simulink model "CryoDetMultiChan_CMB"  (R2016b)
settings: Solver=ode45  StartTime=0.0  StopTime=1000e-6  MaxStep=Tclk/4  RelTol=1e-3
values from neighbouring files (symbols this model uses):
  ds_axi = 16    [setupCryoFPGA_CMB.m]
  Fclk = Fadc    (= 307200000)    [setupCryoFPGA.m]    (also in setupCryoFPGA_CMB.m; setupCryoFPGAorig.m = 312500000)
  notch = tf( [1 a*wNotch/Q wNotch^2], [1 wNotch/Q wNotch^2])    [setupCryoFPGA.m]    (also in setupCryoFPGA_CMB.m; setupCryoFPGAorig.m)
  notch2 = tf( [1 a*wNotch/Q wNotch^2], [1 wNotch/Q wNotch^2])    [setupCryoFPGA.m]    (also in setupCryoFPGA_CMB.m; setupCryoFPGAorig.m)
  notch3 = tf( [1 a*wNotch/Q wNotch^2], [1 wNotch/Q wNotch^2])    [setupCryoFPGA.m]    (also in setupCryoFPGA_CMB.m; setupCryoFPGAorig.m)
  notch4 = tf( [1 a*wNotch/Q wNotch^2], [1 wNotch/Q wNotch^2])    [setupCryoFPGA.m]    (also in setupCryoFPGA_CMB.m; setupCryoFPGAorig.m)
  Tclk = 1/Fclk    (= 3.25520833333e-09)    [setupCryoFPGA.m]    (also in setupCryoFPGA_CMB.m; setupCryoFPGAorig.m = 3.2e-09)
  Ts = 1/Fadc    (= 3.25520833333e-09)    [setupCryoFPGA.m]    (also in setupCryoFPGA_CMB.m; setupCryoFPGAorig.m = 3.2e-09)
undefined symbols (not defined in the file or in its folder): AXI4, i, Lite, xlipgetpartsetting
libraries: xbsIndex_r4 x2077, CryoDetLib x32, hdlsllib x6, simulink x3
(part 1 of 15)
settings Model: Creator=ssmith  LastModifiedBy=jedu
settings DataIOCC: LimitDataPoints=on  SaveFormat=Array
settings OptimizationCC: BlockReduction=off  BooleanDataType=off  LifeSpan=inf
settings DebuggingCC: SaveWithParameterizedLinksMsg=none  UnderspecifiedInitializationDetection=Classic  MergeDetectMultiDrivingBlocksExec=none  SignalResolutionControl=TryResolveAllWithWarning  AllowSymbolicDim=off  SFUnexpectedBacktrackingDiag=warning  SFNoUnconditionalDefaultTransitionDiag=warning  SFExecutionAtInitializationDiag=none
settings HardwareCC: ProdBitPerPointer=32  ProdBitPerSizeT=32  ProdBitPerPtrDiffT=32  ProdLargestAtomicFloat=None  ProdIntDivRoundTo=Undefined  ProdEndianess=Unspecified  ProdWordSize=32  ProdHWDeviceType=32-bit Generic  TargetUnknown=on
settings ModelReferenceCC: PropagateSignalLabelsOutOfModel=off
settings GRTTargetCC: TargetLangStandard=C89/C90 (ANSI)  GeneratePreprocessorConditionals=Disable all
settings ConfigComp: CovMetricSettings=dw  CovHtmlReporting=on  CovSaveCumulativeToWorkspaceVar=on  CovSaveSingleToWorkspaceVar=on  CovExternalEMLEnable=off  CovSFcnEnable=off

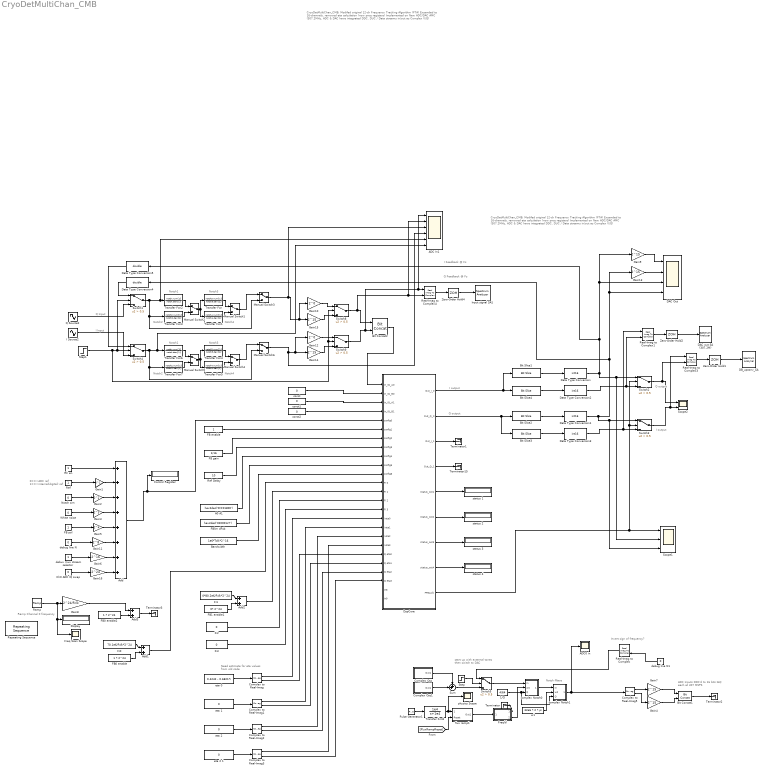
== system CryoDetMultiChan_CMB ==
  note: Notch1
  note: 0==>ADC ref
      | 1==>internal(digital) ref
  note: Q output
  note: I output
  note: Q output
  note: I output
  note: Q Feedback @ Fs
  note: I Feedback @ Fs
  note: Need estimate for eta values
      | from old code
  note: Invert sign of frequency?
  note: Notch filters
  note: start up with external tones
      | then switch to DAC
  note: CryoDetMultiChan_CMB:
      |
      | Modifed original 12-ch Frequency Tracking Algorithm (FTA)
      | Expanded to 16-channels, removed eta calculation (now prog registers)
      | Implemented on New ADC/DAC AMC (307.2MHz, ADC & DAC have integrated DDC, DUC / Data streams in/out as Complex (I/Q)
  note: ADC Inputs DDC'd to
      | 16 bits I&Q each at 307 MSPS
  note: Q Input
  note: I Input
  note: Notch2
  note: Notch3
  note: Notch4
  note: Notch1
  note: Notch2
  note: Notch3
  note: Notch4
  note: Ramp Channel 0 frequency
  note: CryoDetMultiChan_CMB:
      |
      | Modifed original 12-ch Frequency Tracking Algorithm (FTA)
      | Expanded to 16-channels, removed eta calculation (now prog registers)
      | Implemented on New ADC/DAC AMC (307.2MHz, ADC & DAC have integrated DDC, DUC / Data streams in/out as Complex (I/Q)
  1/Q : Constant  Value=4/64  SampleTime=Tclk
  A0 A1 : Constant  Value=hex2dec('FFF01800')  SampleTime=Tclk
  ADC In1 : Scope  NumInputPorts=6
  ADC0 in : Scope
  Add : Sum  Inputs=++++++++
  Add1 : Sum
  Add2 : Sum
  Add3 : Sum
  Bandwidth : Constant  Value=1e6*Tclk*2^16  SampleTime=Tclk
  Bit Concat1 : hdlsllib/HDL Operations/Bit Concat  numInputs=2
  Bit Concat2 : hdlsllib/HDL Operations/Bit Concat  numInputs=2
  Bit Slice1 : hdlsllib/HDL Operations/Bit Slice  lidx=31  ridx=16
  Bit Slice2 : hdlsllib/HDL Operations/Bit Slice  lidx=31  ridx=16
  Bit Slice3 : hdlsllib/HDL Operations/Bit Slice  lidx=15  ridx=0
  Bit Slice4 : hdlsllib/HDL Operations/Bit Slice  lidx=15  ridx=0
  Ch0 ADC IQ swap : Constant  Value=0  SampleTime=Tclk
  Complex Osc : Subsystem  mask{Freq=40e6, Ampl=0.2}
  Complex Osc1 : Subsystem  mask{Freq=50e6, Ampl=0.2}
  Complex to Real-Imag{,1..3,5} (5 alike) : ComplexToRealImag
  Control Register : Display
      settings: Format=decimal (Stored Integer)  Decimation=1000
  DAC Out : Scope  NumInputPorts=4
  DAC out SA (307.2M) : SpectrumAnalyzer
  DB_upconv_SA : SpectrumAnalyzer
  Data Type Conversion{,1..3} (4 alike) : DataTypeConversion  OutDataTypeStr=int16
  Data Type Conversion4 : DataTypeConversion  OutMin=[-0.999]  OutMax=[0.999]  OutDataTypeStr=double  RndMeth=Nearest
  Data Type Conversion5 : DataTypeConversion  OutMin=[-0.999]  OutMax=[0.999]  OutDataTypeStr=double  RndMeth=Nearest
  Display : Display
      settings: Decimation=64
  DspCore : Subsystem
  FB enable : Constant  SampleTime=Tclk
  FB gain : Constant  Value=1/16  SampleTime=Tclk
  FB pol : Constant  SampleTime=Tclk
  FB0 enable : Constant  Value=1 * 2^24  SampleTime=Tclk
  FB0 enable2 : Constant  Value=1 * 2^24  SampleTime=Tclk
  FB1 enable1 : Constant  Value=0* 2^24  SampleTime=Tclk
  FBlim dFsb : Constant  Value=hex2dec('020001c7')  SampleTime=Tclk
  Fi0 : Constant  Value=70.1e6/Fclk*2^24  SampleTime=Tclk
  Fi1 : Constant  Value=0*80.2e6/Fclk*2^24  SampleTime=Tclk
  Fi2 : Constant  Value=0  SampleTime=Tclk
  Fi3 : Constant  Value=0  SampleTime=Tclk
  Freq Scan Scope : Scope
  "Freq(t) " : Subsystem
  Gain1 : Gain  Gain=2^1
  Gain10 : Gain  Gain=2^0  OutDataTypeStr=int16  RndMeth=Nearest  SaturateOnIntegerOverflow=on
  Gain11 : Gain  Gain=2^8
  Gain12 : Gain  Gain=2^0  OutDataTypeStr=int16  RndMeth=Nearest  SaturateOnIntegerOverflow=on
  Gain{4,7,9,13..15} (6 alike) : Gain  Gain=2^15  OutDataTypeStr=int16  RndMeth=Nearest  SaturateOnIntegerOverflow=on
  Gain16 : Gain  Gain=2^24
  Gain2 : Gain  Gain=2^2
  Gain3 : Gain  Gain=2^3
  Gain5 : Gain  Gain=2^4
  Gain6 : Gain  Gain=2^16
  Gain8 : Gain  Gain=2^24/Fclk
  I Source2 : Sin  Amplitude=.999  Frequency=2*pi*70.1e6  Phase=pi/2  SampleTime=0
  Input signal SA1 : SpectrumAnalyzer
  Manual Switch{1..6} (6 alike) : ManualSwitch
  Notch sim : Constant  Value=0  SampleTime=Tclk
  Pulse Generator1 : DiscretePulseGenerator  PulseType=Time based  Amplitude=10  Period=1e-3  PhaseDelay=12e-6
  Q Source2 : Sin  Amplitude=-0.999  Frequency=2*pi*70.1e6  SampleTime=0
  RF en : Constant  SampleTime=Tclk
  Ramp : simulink/Sources/Ramp  slope=1e6/4e-6  start=0  X0=65.1e6
  Real-Imag to Complex{,1,3..4} (4 alike) : RealImagToComplex
  Ref : Constant  SampleTime=Tclk
  Ref Delay : Constant  Value=10  SampleTime=Tclk
  Repeating Sequence : simulink/Sources/Repeating Sequence  rep_seq_t="[0   5e-6  5.1e-6  8e-6 8.1e-6   11e-6 11.1e-6   14e-6 14.1e-6   17e-6 17.1e-6 20e-6 20.1e-6 23e-6 ]"  rep_seq_y="[39.24 39.24 39.49  39.49 39.64 39.64 39.74 39.74 39.84 39.84 39.99 39.99 40.24 40.24]*1e6"
  Scope1 : Scope  NumInputPorts=3
  Scope2 : Scope  NumInputPorts=2
  Step : Step  Time=2e-7  SampleTime=0
  Step1 : Step  Time=200e-9  SampleTime=0
  Sum : Sum  Inputs=++|
  Switch{1..5,8..9} (7 alike) : Switch  Criteria=u2 > Threshold  Threshold=0.5
  Terminator{,1..3,15} (5 alike) : Terminator
  Transfer Fcn : TransferFcn  Numerator=notch3.num{1}  Denominator=notch3.den{1}
  Transfer Fcn1 : TransferFcn  Numerator=notch4.num{1}  Denominator=notch4.den{1}
  Transfer Fcn2 : TransferFcn  Numerator=notch.num{1}  Denominator=notch.den{1}
  Transfer Fcn3 : TransferFcn  Numerator=notch2.num{1}  Denominator=notch2.den{1}
  Transfer Fcn4 : TransferFcn  Numerator=notch3.num{1}  Denominator=notch3.den{1}
  Transfer Fcn5 : TransferFcn  Numerator=notch4.num{1}  Denominator=notch4.den{1}
  Transfer Fcn6 : TransferFcn  Numerator=notch.num{1}  Denominator=notch.den{1}
  Transfer Fcn7 : TransferFcn  Numerator=notch2.num{1}  Denominator=notch2.den{1}
  Transfer Fcn8 : TransferFcn  Numerator=[1e4]  Denominator=[1 1e4]
  White noise : Constant  Value=0  SampleTime=Tclk
  Zero-Order Hold1 : ZeroOrderHold  SampleTime=Ts/2
  Zero-Order Hold2 : ZeroOrderHold  SampleTime=-1
  Zero-Order Hold4 : ZeroOrderHold  SampleTime=Ts
  complex Notch0 : Subsystem
  complex Notch1 : Subsystem
  const : Constant  Value=0  SampleTime=Tclk
  const1 : Constant  Value=0  SampleTime=Tclk
  const2 : Constant  Value=0  SampleTime=Tclk
  debug line N : Constant  Value=0  SampleTime=Tclk
  debug line N1 : Constant  Value=0  SampleTime=Tclk
  debux mux stream selector : Constant  SampleTime=Tclk
  eta 0 : Constant  Value=0.4242 - 0.6821*i
  eta 1 : Constant  Value=0
  "eta 2 " : Constant  Value=0
  eta 2 1 : Constant  Value=0
  flux ramp1 : Subsystem
  physics Scope : Scope
  status {1..4} (4 alike) : Display
  w1 : Constant  Value=32e6 * 2 * pi  SampleTime=Tclk
  wires:
  Add/1 -> DspCore/5(config0), Control Register/1
  FB enable/1 -> DspCore/6(config1)
  RF en/1 -> Add/1
  Ref/1 -> Gain1/1
  Notch sim/1 -> Gain2/1
  White noise/1 -> Gain3/1
  FB pol/1 -> Gain5/1
  Gain1/1 -> Add/2
  Gain2/1 -> Add/3
  Gain3/1 -> Add/4
  Gain5/1 -> Add/5
  FB gain/1 -> DspCore/7(config2)
  Ref Delay/1 -> DspCore/8(config3)
  A0 A1/1 -> DspCore/9(config4)
  FBlim dFsb/1 -> DspCore/10(config5)
  Bandwidth/1 -> DspCore/11(config6)
  Add2/1 -> DspCore/13(Fi 1)
  FB1 enable1/1 -> Add2/2
  Fi1/1 -> Add2/1
  DspCore/9(FPGAclk) -> Switch3/2, Switch2/2, Scope1/1
  DspCore/1(Out_I_0) -> Bit Slice1/1, Bit Slice4/1
  Data Type Conversion1/1 -> Data Type Conversion4/1, DAC Out/4, Gain13/1, Scope1/3, Switch3/1
  Data Type Conversion/1 -> Data Type Conversion5/1, DAC Out/3, Gain9/1, Scope1/2, Switch2/1
  DspCore/2(Out_Q_0) -> Bit Slice3/1, Bit Slice2/1
  Switch2/1 -> Real-Imag to Complex3/2, Scope2/1
  Zero-Order Hold1/1 -> DB_upconv_SA/1
  Real-Imag to Complex3/1 -> Zero-Order Hold1/1
  Bit Slice4/1 -> Data Type Conversion2/1
  Bit Slice3/1 -> Data Type Conversion3/1
  Data Type Conversion2/1 -> Real-Imag to Complex1/2, Switch2/3
  Data Type Conversion3/1 -> Real-Imag to Complex1/1, Switch3/3
  Zero-Order Hold2/1 -> DAC out SA (307.2M)/1
  Real-Imag to Complex1/1 -> Zero-Order Hold2/1
  Switch3/1 -> Real-Imag to Complex3/1, Scope2/2
  DspCore/5(status_out1) -> status 1/1
  DspCore/6(status_out2) -> status 2/1
  DspCore/7(status_out3) -> status 3/1
  DspCore/8(status_out4) -> status 4/1
  eta 1/1 -> Complex to Real-Imag1/1
  "eta 2 "/1 -> Complex to Real-Imag2/1
  Fi2/1 -> DspCore/14(Fi 2)
  Fi3/1 -> DspCore/15(Fi 3)
  Complex to Real-Imag/1 -> DspCore/16(I eta0)
  Complex to Real-Imag/2 -> DspCore/20(Q eta0)
  Complex to Real-Imag1/1 -> DspCore/17(I eta1)
  Complex to Real-Imag1/2 -> DspCore/21(Q eta1)
  eta 2 1/1 -> Complex to Real-Imag3/1
  DspCore/3(Out_I_1) -> Terminator1/1
  DspCore/4(Out_Q_1) -> Terminator15/1
  Complex to Real-Imag2/1 -> DspCore/18(I eta2)
  Complex to Real-Imag2/2 -> DspCore/22(Q eta2)
  Complex to Real-Imag3/1 -> DspCore/19(I eta3)
  Complex to Real-Imag3/2 -> DspCore/23(Q eta3)
  const/1 -> DspCore/2(In_IQ_B0)
  const1/1 -> DspCore/3(In_IQ_A1)
  const2/1 -> DspCore/4(In_IQ_B1)
  Sum/1 -> Switch5/3
  Step/1 -> Switch5/2
  complex Notch1/1(Out) -> Complex to Real-Imag5/1, ADC0 in/1
  Switch5/1 -> complex Notch0/1(In)
  Complex Osc1/1(Out1) -> Sum/2
  Complex Osc/1(Out1) -> Sum/1
  complex Notch0/1(Out) -> complex Notch1/1(In)
  "Freq(t) "/2(omega Out) -> complex Notch0/2(w0)
  w1/1 -> complex Notch1/2(w0)
  1/Q/1 -> complex Notch1/3(Q), complex Notch0/3(Q)
  flux ramp1/1(Out1) -> "Freq(t) "/1(freq in)
  "Freq(t) "/1(Freq Out) -> Terminator/1
  [FluxRampReset] -> flux ramp1/2(Reset)
  Pulse Generator1/1 -> Transfer Fcn8/1
  Transfer Fcn8/1 -> physics Scope/1, flux ramp1/1(physics)
  Real-Imag to Complex/1 -> Switch5/1
  Gain7/1 -> Bit Concat1/1
  Gain4/1 -> Bit Concat1/2
  Complex to Real-Imag5/1 -> Gain7/1
  Complex to Real-Imag5/2 -> Gain4/1
  Manual Switch1/1 -> Manual Switch3/1
  Transfer Fcn1/1 -> Manual Switch1/2
  Transfer Fcn/1 -> Manual Switch1/1
  Transfer Fcn3/1 -> Manual Switch2/2
  Transfer Fcn2/1 -> Manual Switch2/1
  Switch1/1 -> ADC In1/5, Transfer Fcn2/1, Manual Switch3/2, Transfer Fcn3/1
  Manual Switch2/1 -> Transfer Fcn/1, Transfer Fcn1/1
  Step1/1 -> Switch9/2, Switch8/2, Switch4/2, Switch1/2
  Manual Switch4/1 -> Manual Switch6/1
  Transfer Fcn5/1 -> Manual Switch4/2
  Transfer Fcn4/1 -> Manual Switch4/1
  Transfer Fcn7/1 -> Manual Switch5/2
  Transfer Fcn6/1 -> Manual Switch5/1
  Switch4/1 -> ADC In1/6, Transfer Fcn6/1, Manual Switch6/2, Transfer Fcn7/1
  Manual Switch5/1 -> Transfer Fcn4/1, Transfer Fcn5/1
  Manual Switch3/1 -> ADC In1/3, Gain10/1, Gain15/1
  Manual Switch6/1 -> ADC In1/4, Gain12/1, Gain14/1
  Q Source2/1 -> Switch1/3
  I Source2/1 -> Switch4/3
  Bit Concat1/1 -> Terminator2/1
  debug line N1/1 -> Real-Imag to Complex/2
  FB0 enable2/1 -> Add3/2
  Gain8/1 -> Add3/1
  Ramp/1 -> Freq Scan Scope/1, Display/1, Gain8/1
  FB0 enable/1 -> Add1/2
  Fi0/1 -> Add1/1
  Gain9/1 -> DAC Out/1
  Gain13/1 -> DAC Out/2
  Data Type Conversion4/1 -> Switch1/1
  Data Type Conversion5/1 -> Switch4/1
  Zero-Order Hold4/1 -> Input signal SA1/1
  Real-Imag to Complex4/1 -> Zero-Order Hold4/1
  Switch8/1 -> ADC In1/2, Real-Imag to Complex4/2, Bit Concat2/1
  Switch9/1 -> ADC In1/1, Real-Imag to Complex4/1, Bit Concat2/2
  Gain15/1 -> Switch8/3
  Gain14/1 -> Switch9/3
  Bit Concat2/1 -> DspCore/1(In_IQ_A0)
  Gain10/1 -> Switch8/1
  Gain12/1 -> Switch9/1
  Bit Slice1/1 -> Data Type Conversion/1
  Bit Slice2/1 -> Data Type Conversion1/1
  eta 0/1 -> Complex to Real-Imag/1
  Add1/1 -> DspCore/12("Fi 0 ")
  Ch0 ADC IQ swap/1 -> Gain16/1
  debux mux stream selector/1 -> Gain6/1
  debug line N/1 -> Gain11/1
  Gain11/1 -> Add/6
  Gain6/1 -> Add/7
  Gain16/1 -> Add/8
  Add3/1 -> Terminator3/1

== system CryoDetMultiChan_CMB/Complex Osc ==
  Cosine : Sin  Amplitude=Ampl  Frequency=2*pi*Freq  Phase=pi/2  SampleTime=0
  Real-Imag to Complex : RealImagToComplex
  Sine : Sin  Amplitude=Ampl  Frequency=2*pi*Freq  SampleTime=0
  Out1 : Outport
  wires:
  Real-Imag to Complex/1 -> Out1/1
  Cosine/1 -> Real-Imag to Complex/1
  Sine/1 -> Real-Imag to Complex/2

== system CryoDetMultiChan_CMB/Complex Osc1 ==
  Cosine : Sin  Amplitude=Ampl  Frequency=2*pi*Freq  Phase=pi/2  SampleTime=0
  Real-Imag to Complex : RealImagToComplex
  Sine : Sin  Amplitude=Ampl  Frequency=2*pi*Freq  SampleTime=0
  Out1 : Outport
  wires:
  Real-Imag to Complex/1 -> Out1/1
  Cosine/1 -> Real-Imag to Complex/1
  Sine/1 -> Real-Imag to Complex/2

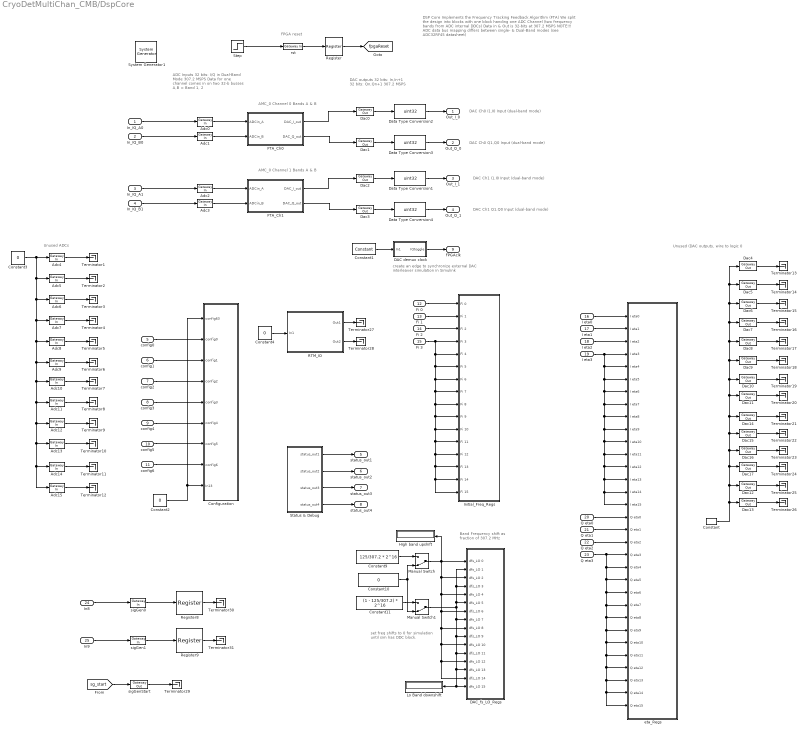
== system CryoDetMultiChan_CMB/DspCore ==
  note: AMC_0 Channel 0
      | Bands A & B
  note: Unused ADCs
  note: create an edge to synchronize external DAC interleaver simulation in Simulink
  note: DAC outputs
      | 32 bits: In,In+1
      | 32 bits: Qn,Qn+1
      | 307.2 MSPS
  note: ADC Inputs
      | 32 bits: I/Q in Dual-Band Mode
      | 307.2 MSPS
      | Data for one channel comes in on two 32-b busses A,B = Band 1, 2
  note: FPGA reset
  note: DAC Ch0 I1,I0 Input (dual-band mode)
  note: DAC Ch0 Q1,Q0 Input (dual-band mode)
  note: DSP Core
      | Implements the Frequency Tracking Feedback Algorithm (FTA)
      | We split the design into blocks with one block handing one ADC Channel
      | (two frequency bands from ADC internal DDCs)
      | Data in & Out is 32-bits at 307.2 MSPS
      |
      | NOTE!!! ADC data bus mapping differs between single- & Dual-Band modes
      | (see ADC32RF45 datasheet)
  note: DAC Ch1 I1,I0 Input (dual-band mode)
  note: DAC Ch1 Q1,Q0 Input (dual-band mode)
  note: Unused (DAC outputs, wire to logic 0
  note: set freq shifts to 0 for simulation
      | until sim has DDC block.
  note: Band Frequency shift as fraction of 307.2 MHz
  note: AMC_0 Channel 1
      | Bands A & B
  In_IQ_A0 : Inport
  In_IQ_B0 : Inport  Port=2
  In_IQ_A1 : Inport  Port=3
  In_IQ_B1 : Inport  Port=4
  config0 : Inport  Port=5
  config1 : Inport  Port=6
  config2 : Inport  Port=7
  config3 : Inport  Port=8
  config4 : Inport  Port=9
  config5 : Inport  Port=10
  config6 : Inport  Port=11
  "Fi 0 " : Inport  Port=12
  Fi 1 : Inport  Port=13
  Fi 2 : Inport  Port=14
  Fi 3 : Inport  Port=15
  I eta0 : Inport  Port=16
  I eta1 : Inport  Port=17
  I eta2 : Inport  Port=18
  I eta3 : Inport  Port=19
  Q eta0 : Inport  Port=20
  Q eta1 : Inport  Port=21
  Q eta2 : Inport  Port=22
  Q eta3 : Inport  Port=23
  In8 : Inport  Port=24
  In9 : Inport  Port=25
  " System Generator1" : xbsIndex_r4/ System Generator  Tag=genX  xilinxfamily=kintexu  part=xcku040  speed=-2-e  package=ffva1156  synthesis_tool=Vivado  clock_wrapper=Clock Enables  directory=./netlist  proj_type=Vivado  Synth_file=Vivado Synthesis Defaults  Impl_file=Vivado Implementation Defaults  testbench=off  simulink_period=Tclk  sysclk_period=Tclk*1e9  dcm_input_clock_period=10  incr_netlist=off  trim_vbits=Everywhere in SubSystem  dbl_ovrd=According to Block Masks  core_generation=According to Block Masks  run_coregen=off  deprecated_control=off  eval_field=0  block_type=sysgen
  Adc{0..15} (16 alike) : xbsIndex_r4/Gateway In  gui_display_data_type=Fixed-point  arith_type=Unsigned  n_bits=32  bin_pt=0  preci_type=Single  exp_width=8  frac_width=24  rows=1  columns=1  quantization=Truncate  overflow=Wrap  period=Ts  UseAsADC=off  ADCChannel='1'  interface=None  automatic_assignment=on  address_offset=hex2dec('00')  intf_name=''  intf_description=''  default_value=0  timing_constraint=None  locs_specified=off  LOCs={}  io_standard={}  inherit_from_input=off  hdl_port=on  dbl_ovrd=off  block_type=gatewayin
  Configuration : Subsystem
  Constant : xbsIndex_r4/Constant  const=0  gui_display_data_type=Fixed-point  arith_type=Signed (2's comp)  n_bits=32  bin_pt=0  preci_type=Single  exp_width=8  frac_width=24  explicit_period=off  period=1  equ=P=C  opselect=C  inp2=PCIN>>17  opr=+  inp1=P  carry=CIN  dbl_ovrd=off  block_type=constant
  Constant1 : xbsIndex_r4/Constant  const=0  gui_display_data_type=Boolean  arith_type=Boolean  n_bits=16  bin_pt=14  preci_type=Single  exp_width=8  frac_width=24  explicit_period=on  period=Tclk  equ=P=C  opselect=C  inp2=PCIN>>17  opr=+  inp1=P  carry=CIN  dbl_ovrd=off  block_type=constant
  Constant{2..4,10} (4 alike) : Constant  Value=0
  Constant11 : Constant  Value=(1 - 125/307.2) * 2^16
  Constant9 : Constant  Value=125/307.2 * 2^16
  DAC demux clock : Subsystem
  DAC_fs_LO_Regs : Subsystem
  Dac{0..17} (18 alike) : xbsIndex_r4/Gateway Out  inherit_from_input=on  hdl_port=on  rows=1  columns=1  UseAsDAC=off  DACChannel='1'  interface=None  automatic_assignment=on  address_offset=hex2dec('00')  intf_name=''  intf_description=''  timing_constraint=None  locs_specified=off  LOCs={}  io_standard={}  block_type=gatewayout
  Data Type Conversion{1..4} (4 alike) : DataTypeConversion  OutDataTypeStr=uint32
  FTA_Ch0 : Subsystem
  FTA_Ch1 : Subsystem
  High band upshift : Display
  Initial_Freq_Regs : Subsystem
  Lo Band downshift : Display
  Manual Switch : ManualSwitch  CurrentSetting=0
  Manual Switch1 : ManualSwitch  CurrentSetting=0
  RTM_IO : Subsystem
  Register : xbsIndex_r4/Register  init=1  rst=off  en=off  dbl_ovrd=off  block_type=register
  Register8 : xbsIndex_r4/Register  init=0  rst=off  en=off  dbl_ovrd=off  block_type=register
  Register9 : xbsIndex_r4/Register  init=0  rst=off  en=off  dbl_ovrd=off  block_type=register
  Status & Debug : Subsystem
  Step : Step  Time=300e-9  Before=1  After=0  SampleTime=0
  Terminator{1..31} (31 alike) : Terminator
  eta_Regs : Subsystem
  rst : xbsIndex_r4/Gateway In  gui_display_data_type=Boolean  arith_type=Boolean  n_bits=16  bin_pt=14  preci_type=Single  exp_width=8  frac_width=24  rows=1  columns=1  quantization="Round  (unbiased: +/- Inf)"  overflow=Saturate  period=Tclk  UseAsADC=off  ADCChannel='1'  interface=None  automatic_assignment=on  address_offset=hex2dec('00')  intf_name=''  intf_description=''  default_value=0  timing_constraint=None  locs_specified=off  LOCs={}  io_standard={}  inherit_from_input=off  hdl_port=on  dbl_ovrd=off  block_type=gatewayin
  sigGen0 : xbsIndex_r4/Gateway In  gui_display_data_type=Fixed-point  arith_type=Unsigned  n_bits=32  bin_pt=0  preci_type=Single  exp_width=8  frac_width=24  rows=1  columns=1  quantization=Truncate  overflow=Wrap  period=Ts  UseAsADC=off  ADCChannel='1'  interface=None  automatic_assignment=on  address_offset=hex2dec('00')  intf_name=''  intf_description=''  default_value=0  timing_constraint=None  locs_specified=off  LOCs={}  io_standard={}  inherit_from_input=off  hdl_port=on  dbl_ovrd=off  block_type=gatewayin
  sigGen1 : xbsIndex_r4/Gateway In  gui_display_data_type=Fixed-point  arith_type=Unsigned  n_bits=32  bin_pt=0  preci_type=Single  exp_width=8  frac_width=24  rows=1  columns=1  quantization=Truncate  overflow=Wrap  period=Ts  UseAsADC=off  ADCChannel='1'  interface=None  automatic_assignment=on  address_offset=hex2dec('00')  intf_name=''  intf_description=''  default_value=0  timing_constraint=None  locs_specified=off  LOCs={}  io_standard={}  inherit_from_input=off  hdl_port=on  dbl_ovrd=off  block_type=gatewayin
  sigGenStart : xbsIndex_r4/Gateway Out  inherit_from_input=on  hdl_port=on  rows=1  columns=1  UseAsDAC=off  DACChannel='1'  interface=None  automatic_assignment=off  address_offset=hex2dec('004')  intf_name=''  intf_description=''  timing_constraint=None  locs_specified=off  LOCs={}  io_standard={}  block_type=gatewayout
  Out_I_0 : Outport
  Out_Q_0 : Outport  Port=2
  Out_I_1 : Outport  Port=3
  Out_Q_1 : Outport  Port=4
  status_out1 : Outport  Port=5
  status_out2 : Outport  Port=6
  status_out3 : Outport  Port=7
  status_out4 : Outport  Port=8
  FPGAclk : Outport  Port=9
  tag scope: fpgaReset=global
  wires:
  In_IQ_A0/1 -> Adc0/1
  Step/1 -> rst/1
  rst/1 -> Register/1
  In_IQ_B0/1 -> Adc1/1
  Adc0/1 -> FTA_Ch0/1(ADCin_A)
  Register/1 -> [fpgaReset]
  Constant2/1 -> Configuration/1(config63), Configuration/9(In13)
  Status & Debug/1(status_out1) -> status_out1/1
  Status & Debug/2(status_out2) -> status_out2/1
  Status & Debug/3(status_out3) -> status_out3/1
  Status & Debug/4(status_out4) -> status_out4/1
  DAC demux clock/1(IQtoggle) -> FPGAclk/1
  Dac1/1 -> Data Type Conversion3/1
  FTA_Ch0/1(DAC_I_out) -> Dac0/1
  FTA_Ch0/2(DAC_Q_out) -> Dac1/1
  Data Type Conversion2/1 -> Out_I_0/1
  Dac0/1 -> Data Type Conversion2/1
  Data Type Conversion3/1 -> Out_Q_0/1
  config0/1 -> Configuration/2(config0)
  config1/1 -> Configuration/3(config1)
  config2/1 -> Configuration/4(config2)
  config4/1 -> Configuration/6(config4)
  config5/1 -> Configuration/7(config5)
  config6/1 -> Configuration/8(config6)
  In_IQ_B1/1 -> Adc3/1
  In_IQ_A1/1 -> Adc2/1
  Adc1/1 -> FTA_Ch0/2(ADCin_B)
  Adc2/1 -> FTA_Ch1/1(ADCin_A)
  Adc3/1 -> FTA_Ch1/2(ADCin_B)
  Adc4/1 -> Terminator1/1
  Adc5/1 -> Terminator2/1
  Adc6/1 -> Terminator3/1
  Adc7/1 -> Terminator4/1
  Adc8/1 -> Terminator5/1
  Adc9/1 -> Terminator6/1
  Adc10/1 -> Terminator7/1
  Adc11/1 -> Terminator8/1
  Adc12/1 -> Terminator9/1
  Adc13/1 -> Terminator10/1
  Adc14/1 -> Terminator11/1
  Adc15/1 -> Terminator12/1
  Dac3/1 -> Data Type Conversion4/1
  FTA_Ch1/1(DAC_I_out) -> Dac2/1
  FTA_Ch1/2(DAC_Q_out) -> Dac3/1
  Dac2/1 -> Data Type Conversion1/1
  Data Type Conversion1/1 -> Out_I_1/1
  Data Type Conversion4/1 -> Out_Q_1/1
  config3/1 -> Configuration/5(config3)
  Constant/1 -> Dac13/1, Dac12/1, Dac17/1, Dac16/1, Dac15/1, Dac14/1, Dac11/1, Dac10/1, Dac8/1, Dac7/1, Dac6/1, Dac5/1, Dac4/1, Dac9/1
  "Fi 0 "/1 -> Initial_Freq_Regs/1("Fi 0 ")
  Fi 1/1 -> Initial_Freq_Regs/2(Fi 1)
  Fi 2/1 -> Initial_Freq_Regs/3(Fi 2)
  Fi 3/1 -> Initial_Freq_Regs/5(Fi 4), Initial_Freq_Regs/6(Fi 5), Initial_Freq_Regs/7(Fi 6), Initial_Freq_Regs/8(Fi 7), Initial_Freq_Regs/9(Fi 8), Initial_Freq_Regs/10(Fi 9), Initial_Freq_Regs/11(Fi 10), Initial_Freq_Regs/12(Fi 11), Initial_Freq_Regs/13(Fi 12), Initial_Freq_Regs/14(Fi 13), Initial_Freq_Regs/15(Fi 14), Initial_Freq_Regs/16(Fi 15), Initial_Freq_Regs/4(Fi 3)
  I eta0/1 -> eta_Regs/1("I eta0 ")
  I eta1/1 -> eta_Regs/2(I eta1)
  I eta2/1 -> eta_Regs/3(I eta2)
  Q eta0/1 -> eta_Regs/17(Q eta0)
  Q eta1/1 -> eta_Regs/18(Q eta1)
  Q eta2/1 -> eta_Regs/19(Q eta2)
  Dac4/1 -> Terminator13/1
  Constant3/1 -> Adc5/1, Adc6/1, Adc7/1, Adc8/1, Adc9/1, Adc10/1, Adc11/1, Adc12/1, Adc13/1, Adc14/1, Adc15/1, Adc4/1
  Dac5/1 -> Terminator14/1
  Dac6/1 -> Terminator15/1
  Dac7/1 -> Terminator16/1
  Dac8/1 -> Terminator17/1
  Dac9/1 -> Terminator18/1
  Dac10/1 -> Terminator19/1
  Dac11/1 -> Terminator20/1
  Dac14/1 -> Terminator21/1
  Dac15/1 -> Terminator22/1
  Dac16/1 -> Terminator23/1
  Dac17/1 -> Terminator24/1
  Dac12/1 -> Terminator25/1
  Dac13/1 -> Terminator26/1
  Manual Switch/1 -> DAC_fs_LO_Regs/1("dfs_LO 0 "), DAC_fs_LO_Regs/3(dfs_LO 2), DAC_fs_LO_Regs/5(dfs_LO 4), DAC_fs_LO_Regs/7(dfs_LO 6), DAC_fs_LO_Regs/9(dfs_LO 8), DAC_fs_LO_Regs/11(dfs_LO 10), DAC_fs_LO_Regs/13(dfs_LO 12), DAC_fs_LO_Regs/15(dfs_LO 14), High band upshift/1
  Constant9/1 -> Manual Switch/1
  Constant10/1 -> Manual Switch/2, Manual Switch1/2
  Constant11/1 -> Manual Switch1/1
  Manual Switch1/1 -> DAC_fs_LO_Regs/8(dfs_LO 7), DAC_fs_LO_Regs/10(dfs_LO 9), DAC_fs_LO_Regs/12(dfs_LO 11), DAC_fs_LO_Regs/14(dfs_LO 13), DAC_fs_LO_Regs/16(dfs_LO 15), Lo Band downshift/1, DAC_fs_LO_Regs/6(dfs_LO 5), DAC_fs_LO_Regs/4(dfs_LO 3), DAC_fs_LO_Regs/2(dfs_LO 1)
  I eta3/1 -> eta_Regs/5(I eta4), eta_Regs/6(I eta5), eta_Regs/7(I eta6), eta_Regs/8(I eta7), eta_Regs/9(I eta8), eta_Regs/10(I eta9), eta_Regs/11(I eta10), eta_Regs/12(I eta11), eta_Regs/13(I eta12), eta_Regs/14(I eta13), eta_Regs/15(I eta14), eta_Regs/16(I eta15), eta_Regs/4(I eta3)
  Q eta3/1 -> eta_Regs/21(Q eta4), eta_Regs/22(Q eta5), eta_Regs/23(Q eta6), eta_Regs/24(Q eta7), eta_Regs/25(Q eta8), eta_Regs/26(Q eta9), eta_Regs/27(Q eta10), eta_Regs/28(Q eta11), eta_Regs/29(Q eta12), eta_Regs/30(Q eta13), eta_Regs/31(Q eta14), eta_Regs/32(Q eta15), eta_Regs/20(Q eta3)
  Constant4/1 -> RTM_IO/1(In1)
  RTM_IO/1(Out1) -> Terminator27/1
  RTM_IO/2(Out2) -> Terminator28/1
  Constant1/1 -> DAC demux clock/1(In1)
  In8/1 -> sigGen0/1
  sigGen0/1 -> Register8/1
  In9/1 -> sigGen1/1
  sigGen1/1 -> Register9/1
  sigGenStart/1 -> Terminator29/1
  [sg_start] -> sigGenStart/1
  Register8/1 -> Terminator30/1
  Register9/1 -> Terminator31/1

== system CryoDetMultiChan_CMB/Freq(t)  ==
  freq in : Inport
  Afm : Constant  Value=0.25e6
  Gain : Gain  Gain=2*pi
  Product : Product
  Ramp 0-1 : simulink/Sources/Repeating Sequence  rep_seq_t=[0 100e-6]  rep_seq_y=[0 1]
  Sine Wave Function : Sin  TimeSource=Use external signal  Frequency=2*pi  SampleTime=0
  Sum1 : Sum  Inputs=++|
  Freq Out : Outport
  omega Out : Outport  Port=2
  wires:
  Sum1/1 -> Gain/1, Freq Out/1
  Product/1 -> Sine Wave Function/1
  Ramp 0-1/1 -> Product/1
  Afm/1 -> Product/2
  Gain/1 -> omega Out/1
  Sine Wave Function/1 -> Sum1/2
  freq in/1 -> Sum1/1

== system CryoDetMultiChan_CMB/complex Notch0 ==
  In : Inport
  w0 : Inport  Port=2
  Q : Inport  Port=3
  Complex to Real-Imag : ComplexToRealImag
  Real-Imag to Complex : RealImagToComplex
  imNotch : Subsystem
  reNotch : Subsystem
  Out : Outport
  wires:
  w0/1 -> reNotch/2(w0), imNotch/2(w0)
  In/1 -> Complex to Real-Imag/1
  Q/1 -> imNotch/3(1/Q), reNotch/3(1/Q)
  Complex to Real-Imag/1 -> reNotch/1(In)
  reNotch/1(outt) -> Real-Imag to Complex/1
  imNotch/1(outt) -> Real-Imag to Complex/2
  Complex to Real-Imag/2 -> imNotch/1(In)
  Real-Imag to Complex/1 -> Out/1

== system CryoDetMultiChan_CMB/complex Notch1 ==
  In : Inport
  w0 : Inport  Port=2
  Q : Inport  Port=3
  Complex to Real-Imag : ComplexToRealImag
  Real-Imag to Complex : RealImagToComplex
  imNotch : Subsystem
  reNotch : Subsystem
  Out : Outport
  wires:
  w0/1 -> reNotch/2(w0), imNotch/2(w0)
  In/1 -> Complex to Real-Imag/1
  Q/1 -> imNotch/3(1/Q), reNotch/3(1/Q)
  Complex to Real-Imag/1 -> reNotch/1(In)
  reNotch/1(outt) -> Real-Imag to Complex/1
  imNotch/1(outt) -> Real-Imag to Complex/2
  Complex to Real-Imag/2 -> imNotch/1(In)
  Real-Imag to Complex/1 -> Out/1

== system CryoDetMultiChan_CMB/flux ramp1 ==
  note: Simulate flux-ramp modulated center frequency of notch
      | with reset from flux ramp reset
  physics : Inport
  Reset : Inport  Port=2
  Add : Sum  Inputs=++|
  Add4 : Sum
  F1 : Constant  Value=0 * 307.2e6 / 16 / 16
  F3 : Constant  Value=64e6
  Integrator : Integrator  ExternalReset=rising
  Resonator w Flux Ramp Scope : Scope
  Resonator w Flux Ramp Scope1 : Scope
  Sine Wave : Sin  TimeSource=Use external signal  Amplitude=0.1e6  Frequency=2*pi  SampleTime=0
  Out1 : Outport
  wires:
  Add4/1 -> Resonator w Flux Ramp Scope/1, Out1/1
  F3/1 -> Add4/2
  F1/1 -> Integrator/1
  Reset/1 -> Integrator/2
  Sine Wave/1 -> Add4/1
  Integrator/1 -> Add/2
  Add/1 -> Resonator w Flux Ramp Scope1/1, Sine Wave/1
  physics/1 -> Add/1

== system CryoDetMultiChan_CMB/DspCore/Configuration ==
  note: Frequencies in phase increment per clock
      | where 2^16 = 2 pi
  note: initial frequencies
  note: Configuration Registers
  note: Command Register
  note: Break out bits from Control Register (Config reg 0)
  note: Bandwidth in phase increment per clock
      | where 2^16 = 2 pi e.g 4.6875KHz/count
  config63 : Inport
  config0 : Inport  Port=2
  config1 : Inport  Port=3
  config2 : Inport  Port=4
  config3 : Inport  Port=5
  config4 : Inport  Port=6
  config5 : Inport  Port=7
  config6 : Inport  Port=8
  In13 : Inport  Port=9
  BitBasher : xbsIndex_r4/BitBasher  bitexpr=b={a[24]}  display_expr=off  sr_1=b  arith_type1=Unsigned  bin_pt1=0  sr_2=2  arith_type2=Unsigned  bin_pt2=0  sr_3=3  arith_type3=Unsigned  bin_pt3=0  sr_4=4  arith_type4=Unsigned  bin_pt4=0  dbl_ovrd=off  block_type=bitbasher
  BitBasher1 : xbsIndex_r4/BitBasher  bitexpr=b={a[25]}  display_expr=off  sr_1=b  arith_type1=Unsigned  bin_pt1=0  sr_2=2  arith_type2=Unsigned  bin_pt2=0  sr_3=3  arith_type3=Unsigned  bin_pt3=0  sr_4=4  arith_type4=Unsigned  bin_pt4=0  dbl_ovrd=off  block_type=bitbasher
  BitBasher12 : xbsIndex_r4/BitBasher  bitexpr=a={b[31:16]}  display_expr=on  sr_1=a  arith_type1=Unsigned  bin_pt1=16  sr_2=2  arith_type2=Unsigned  bin_pt2=0  sr_3=3  arith_type3=Unsigned  bin_pt3=0  sr_4=4  arith_type4=Unsigned  bin_pt4=0  dbl_ovrd=off  block_type=bitbasher
  BitBasher15 : xbsIndex_r4/BitBasher  bitexpr=a={b[15:0]}  display_expr=on  sr_1=a  arith_type1=Unsigned  bin_pt1=12  sr_2=2  arith_type2=Unsigned  bin_pt2=0  sr_3=3  arith_type3=Unsigned  bin_pt3=0  sr_4=4  arith_type4=Unsigned  bin_pt4=0  dbl_ovrd=off  block_type=bitbasher
  BitBasher16 : xbsIndex_r4/BitBasher  bitexpr=a={b[15:0]}  display_expr=on  sr_1=a  arith_type1="Signed  (2's comp)"  bin_pt1=15  sr_2=2  arith_type2=Unsigned  bin_pt2=0  sr_3=3  arith_type3=Unsigned  bin_pt3=0  sr_4=4  arith_type4=Unsigned  bin_pt4=0  dbl_ovrd=off  block_type=bitbasher
  BitBasher2 : xbsIndex_r4/BitBasher  bitexpr=b={a[0]}  display_expr=on  sr_1=b  arith_type1=Unsigned  bin_pt1=0  sr_2=2  arith_type2=Unsigned  bin_pt2=0  sr_3=3  arith_type3=Unsigned  bin_pt3=0  sr_4=4  arith_type4=Unsigned  bin_pt4=0  dbl_ovrd=off  block_type=bitbasher
  BitBasher3 : xbsIndex_r4/BitBasher  bitexpr=b={a[0]}  display_expr=on  sr_1=b  arith_type1=Unsigned  bin_pt1=0  sr_2=2  arith_type2=Unsigned  bin_pt2=0  sr_3=3  arith_type3=Unsigned  bin_pt3=0  sr_4=4  arith_type4=Unsigned  bin_pt4=0  dbl_ovrd=off  block_type=bitbasher
  Control Reg : Display
  Convert : xbsIndex_r4/Convert  gui_display_data_type=Boolean  arith_type=Boolean  n_bits=16  bin_pt=14  float_type=Single  exp_bits=8  fraction_bits=24  quantization=Truncate  overflow=Wrap  en=off  latency=1  pipeline=off  dbl_ovrd=off  block_type=convert
  Convert1 : xbsIndex_r4/Convert  gui_display_data_type=Boolean  arith_type=Boolean  n_bits=16  bin_pt=14  float_type=Single  exp_bits=8  fraction_bits=24  quantization=Truncate  overflow=Wrap  en=off  latency=1  pipeline=off  dbl_ovrd=off  block_type=convert
  Convert2 : xbsIndex_r4/Convert  gui_display_data_type=Boolean  arith_type=Boolean  n_bits=16  bin_pt=14  float_type=Single  exp_bits=8  fraction_bits=24  quantization=Truncate  overflow=Wrap  en=off  latency=1  pipeline=off  dbl_ovrd=off  block_type=convert
  Gateway Out6 : xbsIndex_r4/Gateway Out  inherit_from_input=off  hdl_port=off  rows=1  columns=1  UseAsDAC=off  DACChannel='1'  interface=None  automatic_assignment=on  address_offset=hex2dec('00')  intf_name=''  intf_description=''  timing_constraint=None  locs_specified=off  LOCs={}  io_standard={}  block_type=gatewayout
  Register{1..20,22..29} (28 alike) : xbsIndex_r4/Register  init=0  rst=off  en=off  dbl_ovrd=off  block_type=register
  Reinterpret : xbsIndex_r4/Reinterpret  force_arith_type=on  arith_type=Unsigned  force_bin_pt=on  bin_pt=16  block_type=reinterpret
  Slice : xbsIndex_r4/Slice  nbits=1  boolean_output=on  mode=Lower Bit Location + Width  bit1=0  base1=LSB of Input  bit0=0  base0=LSB of Input  dbl_ovrd=off  block_type=slice
  Slice1 : xbsIndex_r4/Slice  nbits=1  boolean_output=on  mode=Upper Bit Location + Width  bit1=1  base1=LSB of Input  bit0=0  base0=LSB of Input  dbl_ovrd=off  block_type=slice
  Slice14 : xbsIndex_r4/Slice  nbits=8  boolean_output=off  mode=Lower Bit Location + Width  bit1=0  base1=LSB of Input  bit0=0  base0=LSB of Input  dbl_ovrd=off  block_type=slice
  Slice2 : xbsIndex_r4/Slice  nbits=1  boolean_output=on  mode=Upper Bit Location + Width  bit1=2  base1=LSB of Input  bit0=0  base0=LSB of Input  dbl_ovrd=off  block_type=slice
  Slice5 : xbsIndex_r4/Slice  nbits=16  boolean_output=off  mode=Upper Bit Location + Width  bit1=31  base1=LSB of Input  bit0=0  base0=LSB of Input  dbl_ovrd=off  block_type=slice
  Slice7 : xbsIndex_r4/Slice  nbits=1  boolean_output=on  mode=Upper Bit Location + Width  bit1=4  base1=LSB of Input  bit0=0  base0=LSB of Input  dbl_ovrd=off  block_type=slice
  Slice8 : xbsIndex_r4/Slice  nbits=8  boolean_output=off  mode=Lower Bit Location + Width  bit1=6  base1=LSB of Input  bit0=16  base0=LSB of Input  dbl_ovrd=off  block_type=slice
  Slice9 : xbsIndex_r4/Slice  nbits=8  boolean_output=off  mode=Lower Bit Location + Width  bit1=6  base1=LSB of Input  bit0=8  base0=LSB of Input  dbl_ovrd=off  block_type=slice
  Terminator1 : Terminator
  Terminator16 : Terminator
  Terminator2 : Terminator
  Up Sample : xbsIndex_r4/Up Sample  sample_ratio=8  copy_samples=off  en=off  latency=1  dbl_ovrd=off  block_type=usamp
  fromDsp_status511 : xbsIndex_r4/Gateway Out  inherit_from_input=on  hdl_port=on  rows=1  columns=1  UseAsDAC=off  DACChannel='1'  interface=AXI4-Lite  automatic_assignment=off  address_offset=hex2dec('7FC')  intf_name=''  intf_description=''  timing_constraint=None  locs_specified=off  LOCs={}  io_standard={}  block_type=gatewayout
  toDsp_cmd0 : xbsIndex_r4/Gateway In  gui_display_data_type=Fixed-point  arith_type=Unsigned  n_bits=32  bin_pt=0  preci_type=Single  exp_width=8  frac_width=24  rows=1  columns=1  quantization=Truncate  overflow=Wrap  period=Tclk  UseAsADC=off  ADCChannel='1'  interface=AXI4-Lite  automatic_assignment=off  address_offset=hex2dec('8fc')  intf_name=''  intf_description=''  default_value=0  timing_constraint=None  locs_specified=off  LOCs={}  io_standard={}  inherit_from_input=off  hdl_port=on  dbl_ovrd=off  block_type=gatewayin
  toDsp_config0 : xbsIndex_r4/Gateway In  gui_display_data_type=Fixed-point  arith_type=Unsigned  n_bits=32  bin_pt=0  preci_type=Single  exp_width=8  frac_width=24  rows=1  columns=1  quantization=Truncate  overflow=Wrap  period=Tclk*ds_axi  UseAsADC=off  ADCChannel='1'  interface=AXI4-Lite  automatic_assignment=off  address_offset=hex2dec('800')  intf_name=''  intf_description=''  default_value=0  timing_constraint=None  locs_specified=off  LOCs={}  io_standard={}  inherit_from_input=off  hdl_port=on  dbl_ovrd=off  block_type=gatewayin
  toDsp_config1 : xbsIndex_r4/Gateway In  gui_display_data_type=Fixed-point  arith_type=Unsigned  n_bits=32  bin_pt=0  preci_type=Single  exp_width=8  frac_width=24  rows=1  columns=1  quantization=Truncate  overflow=Wrap  period=Tclk*ds_axi  UseAsADC=off  ADCChannel='1'  interface=AXI4-Lite  automatic_assignment=off  address_offset=hex2dec('804')  intf_name=''  intf_description=''  default_value=0  timing_constraint=None  locs_specified=off  LOCs={}  io_standard={}  inherit_from_input=off  hdl_port=on  dbl_ovrd=off  block_type=gatewayin
  toDsp_config2 : xbsIndex_r4/Gateway In  gui_display_data_type=Fixed-point  arith_type=Unsigned  n_bits=32  bin_pt=12  preci_type=Single  exp_width=8  frac_width=24  rows=1  columns=1  quantization=Truncate  overflow=Wrap  period=Tclk*ds_axi  UseAsADC=off  ADCChannel='1'  interface=AXI4-Lite  automatic_assignment=off  address_offset=hex2dec('808')  intf_name=''  intf_description=''  default_value=0  timing_constraint=None  locs_specified=off  LOCs={}  io_standard={}  inherit_from_input=off  hdl_port=on  dbl_ovrd=off  block_type=gatewayin
  toDsp_config3 : xbsIndex_r4/Gateway In  gui_display_data_type=Fixed-point  arith_type=Unsigned  n_bits=32  bin_pt=0  preci_type=Single  exp_width=8  frac_width=24  rows=1  columns=1  quantization=Truncate  overflow=Wrap  period=Tclk*ds_axi  UseAsADC=off  ADCChannel='1'  interface=AXI4-Lite  automatic_assignment=off  address_offset=hex2dec('80c')  intf_name=''  intf_description=''  default_value=0  timing_constraint=None  locs_specified=off  LOCs={}  io_standard={}  inherit_from_input=off  hdl_port=on  dbl_ovrd=off  block_type=gatewayin
  toDsp_config4 : xbsIndex_r4/Gateway In  gui_display_data_type=Fixed-point  arith_type=Unsigned  n_bits=32  bin_pt=0  preci_type=Single  exp_width=8  frac_width=24  rows=1  columns=1  quantization=Truncate  overflow=Wrap  period=Tclk*ds_axi  UseAsADC=off  ADCChannel='1'  interface=AXI4-Lite  automatic_assignment=off  address_offset=hex2dec('810')  intf_name=''  intf_description=''  default_value=0  timing_constraint=None  locs_specified=off  LOCs={}  io_standard={}  inherit_from_input=off  hdl_port=on  dbl_ovrd=off  block_type=gatewayin
  toDsp_config5 : xbsIndex_r4/Gateway In  gui_display_data_type=Fixed-point  arith_type=Unsigned  n_bits=32  bin_pt=0  preci_type=Single  exp_width=8  frac_width=24  rows=1  columns=1  quantization=Truncate  overflow=Wrap  period=Tclk  UseAsADC=off  ADCChannel='1'  interface=AXI4-Lite  automatic_assignment=off  address_offset=hex2dec('814')  intf_name=''  intf_description=''  default_value=0  timing_constraint=None  locs_specified=off  LOCs={}  io_standard={}  inherit_from_input=off  hdl_port=on  dbl_ovrd=off  block_type=gatewayin
  toDsp_config511 : xbsIndex_r4/Gateway In  gui_display_data_type=Fixed-point  arith_type=Unsigned  n_bits=32  bin_pt=0  preci_type=Single  exp_width=8  frac_width=24  rows=1  columns=1  quantization=Truncate  overflow=Wrap  period=Tclk*ds_axi  UseAsADC=off  ADCChannel='1'  interface=AXI4-Lite  automatic_assignment=off  address_offset=hex2dec('FFC')  intf_name=''  intf_description=''  default_value=0  timing_constraint=None  locs_specified=off  LOCs={}  io_standard={}  inherit_from_input=off  hdl_port=on  dbl_ovrd=off  block_type=gatewayin
  toDsp_config6 : xbsIndex_r4/Gateway In  gui_display_data_type=Fixed-point  arith_type=Unsigned  n_bits=32  bin_pt=0  preci_type=Single  exp_width=8  frac_width=24  rows=1  columns=1  quantization=Truncate  overflow=Wrap  period=Tclk*ds_axi  UseAsADC=off  ADCChannel='1'  interface=AXI4-Lite  automatic_assignment=off  address_offset=hex2dec('818')  intf_name=''  intf_description=''  default_value=0  timing_constraint=None  locs_specified=off  LOCs={}  io_standard={}  inherit_from_input=off  hdl_port=on  dbl_ovrd=off  block_type=gatewayin
  tag scope: Ampl0=global, BW=global, Band1_IQ_In_Swap=global, ConfigReg0=global, FBen=global, FBgain=global, FBlimit=global, FBreset=global, NotchSimEn=global, RFen=global, RefSource=global, debugMux=global, fbPolarity=global, monitorChannel=global, refDel=global, sg_start=global
  wires:
  config0/1 -> toDsp_config0/1
  toDsp_config0/1 -> Register2/1
  config4/1 -> toDsp_config4/1
  toDsp_config4/1 -> Register3/1
  config5/1 -> toDsp_config5/1
  toDsp_config5/1 -> Register4/1
  config63/1 -> toDsp_cmd0/1
  toDsp_cmd0/1 -> Register6/1
  Register6/1 -> Register7/1
  Slice5/1 -> Reinterpret/1
  Register25/1 -> BitBasher12/1
  Register10/1 -> BitBasher2/1, [ConfigReg0], Gateway Out6/1, Slice1/1, Slice2/1, Slice7/1, BitBasher/1, BitBasher1/1, Slice8/1, Slice9/1
  Slice1/1 -> [RefSource]
  BitBasher2/1 -> [RFen]
  Slice2/1 -> [NotchSimEn]
  Reinterpret/1 -> [Ampl0]
  Gateway Out6/1 -> Control Reg/1
  BitBasher3/1 -> Convert1/1
  BitBasher12/1 -> [FBlimit]
  [NotchSimEn] -> Terminator2/1
  Slice9/1 -> [monitorChannel]
  In13/1 -> toDsp_config511/1
  toDsp_config511/1 -> Register11/1
  Register29/1 -> fromDsp_status511/1
  fromDsp_status511/1 -> Terminator16/1
  config1/1 -> toDsp_config1/1
  toDsp_config1/1 -> Register12/1
  config2/1 -> toDsp_config2/1
  toDsp_config2/1 -> Register13/1
  config3/1 -> toDsp_config3/1
  toDsp_config3/1 -> Register14/1
  Slice/1 -> [FBen]
  BitBasher15/1 -> [FBgain]
  Slice14/1 -> [refDel]
  config6/1 -> toDsp_config6/1
  toDsp_config6/1 -> Register15/1
  Register27/1 -> BitBasher16/1
  Slice7/1 -> [fbPolarity]
  [RefSource] -> Terminator1/1
  Slice8/1 -> [debugMux]
  BitBasher16/1 -> [BW]
  BitBasher/1 -> Convert/1
  Convert/1 -> [Band1_IQ_In_Swap]
  Convert1/1 -> [FBreset]
  BitBasher1/1 -> Convert2/1
  Convert2/1 -> [sg_start]
  Up Sample/1 -> Register5/1
  Register5/1 -> Slice14/1
  Register7/1 -> Register8/1
  Register8/1 -> BitBasher3/1
  Register9/1 -> Register10/1
  Register16/1 -> Register17/1
  Register18/1 -> Register19/1
  Register17/1 -> Slice/1
  Register22/1 -> Register23/1
  Register3/1 -> Register22/1
  Register24/1 -> Register25/1
  Register26/1 -> Register27/1
  Register19/1 -> BitBasher15/1
  Register2/1 -> Register9/1
  Register12/1 -> Register16/1
  Register13/1 -> Register18/1
  Register14/1 -> Register20/1
  Register20/1 -> Register1/1
  Register23/1 -> Slice5/1
  Register4/1 -> Register24/1
  Register15/1 -> Register26/1
  Register28/1 -> Register29/1
  Register11/1 -> Register28/1
  Register1/1 -> Up Sample/1

== system CryoDetMultiChan_CMB/DspCore/DAC demux clock ==
  note: Use DAC clock to generate edge to synchronize simulation of DAC demuxing in FPGA VHDL wrapper
      | output 1 = I
      | 0 = Q
      | This generates no code in FPGA, it is just  here to make Simulink simulation run
  In1 : Inport
  Add : Sum
  Clock Enable Probe : xbsIndex_r4/Clock Enable Probe  inherit_constraints=on  block_type=ceprobe
      settings: infoedit="Clock enable extractor.  Produces a Boolean output that mirrors the hardware clock enable associated with the input sample rate.<br><br>Hardware notes: in hardware this block costs nothing."
  Constant : Constant  Value=2
  DAC_dmux_clk Scope : Scope  NumInputPorts=2
  Down Sample : xbsIndex_r4/Down Sample  sample_ratio=2  sample_phase="Last Value of Frame  (most efficient)"  en=off  rst=off  latency=1  dbl_ovrd=off  block_type=dsamp
  Math Function : Math  Operator=mod  SaturateOnIntegerOverflow=on
  Transport Delay : TransportDelay  DelayTime=Tclk/2
  fromdsp_dacdata1_2 : xbsIndex_r4/Gateway Out  inherit_from_input=off  hdl_port=off  rows=1  columns=1  UseAsDAC=off  DACChannel='1'  interface=None  automatic_assignment=on  address_offset=hex2dec('00')  intf_name=''  intf_description=''  timing_constraint=None  locs_specified=off  LOCs={}  io_standard={}  block_type=gatewayout
  IQtoggle : Outport
  wires:
  Clock Enable Probe/1 -> DAC_dmux_clk Scope/2, fromdsp_dacdata1_2/1
  Down Sample/1 -> Clock Enable Probe/1
  In1/1 -> Down Sample/1
  fromdsp_dacdata1_2/1 -> Add/1, Transport Delay/1
  Transport Delay/1 -> Add/2
  Add/1 -> Math Function/1
  Math Function/1 -> DAC_dmux_clk Scope/1, IQtoggle/1
  Constant/1 -> Math Function/2
